simulink model "SimpleCalc_SF_Topic3_Task1"  (R2019a)
settings: Solver=FixedStepDiscrete  StartTime=0.0  StopTime=10.0  RelTol=1e-3
settings Model: Creator=Raouf  LastModifiedBy=Raouf
settings OptimizationCC: DefaultParameterBehavior=Inlined  EnhancedBackFolding=on  PassReuseOutputArgsAs=Individual arguments  OptimizeBlockOrder=speed  DifferentSizesBufferReuse=on  OptimizationCustomize=off
settings DebuggingCC: ParameterTunabilityLossMsg=error
settings SFSimCC: MATLABDynamicMemAlloc=off
settings RTWCC: SystemTargetFile=ert.tlc  GenCodeOnly=on  TemplateMakefile=ert_default_tmf  GenerateReport=on  IncludeHyperlinkInReport=on  LaunchReport=on  GenerateTraceInfo=on  GenerateTraceReport=on  GenerateTraceReportSl=on  GenerateTraceReportSf=on  GenerateTraceReportEml=on
settings CodeAppCC: ForceParamTrailComments=on  IgnoreCustomStorageClasses=off  OperatorAnnotations=on  SimulinkDataObjDesc=on  SFDataObjDesc=on  InsertBlockDesc=on
settings ERTTargetCC: TargetLangStandard=C99 (ISO)  GenerateSampleERTMain=on  InlinedParameterPlacement=NonHierarchical  ERTCustomFileTemplate=example_file_process.tlc

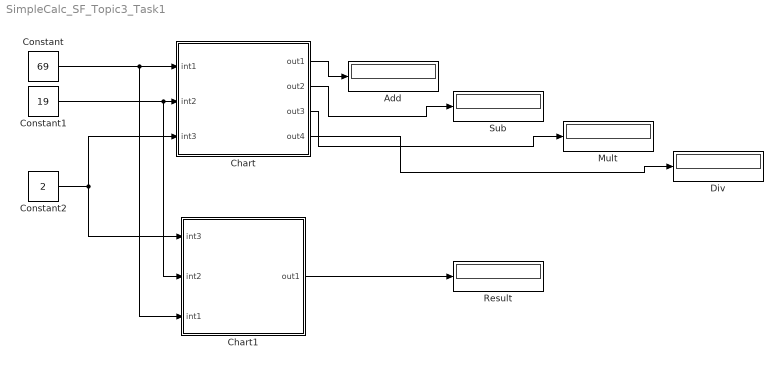
== system SimpleCalc_SF_Topic3_Task1 ==
  Add : Display
  Chart : Stateflow chart  TreatAsAtomicUnit=on
  Chart1 : Stateflow chart  BlockKeywords=__PRM__SERIALIZED__DATA__:Stateflow Chart,Stateflow Diagram  TreatAsAtomicUnit=on
  Constant : Constant  Value=69  OutDataTypeStr=int32
  Constant1 : Constant  Value=19  OutDataTypeStr=int32
  Constant2 : Constant  Value=2  OutDataTypeStr=int32
  Div : Display
  Mult : Display
  Result : Display
  Sub : Display
  wires:
  Chart/1(out1) -> Add/1
  Chart/2(out2) -> Sub/1
  Chart/3(out3) -> Mult/1
  Chart/4(out4) -> Div/1
  Constant/1 -> Chart/1(int1), Chart1/3(int1)
  Constant1/1 -> Chart1/2(int2), Chart/2(int2)
  Constant2/1 -> Chart/3(int3), Chart1/1(int3)
  Chart1/1(out1) -> Result/1

== stateflow chart SimpleCalc_SF_Topic3_Task1/Chart1 ==
  note: Do not put any code along
      | the transitions that run
      | down the right side!
  (default) -> (junction 27) : % calculator
  (junction 27) -> (junction 28) [order 1] : [int3 == 1]
  (junction 27) -> (junction 31) [order 2]
  (junction 28) -> (junction 29) : {out1 = int1 + int2;}
  (junction 29) -> (junction 30)
  (junction 30) -> (junction 34)
  (junction 31) -> (junction 32) [order 1] : [int3 == 2]
  (junction 31) -> (junction 35) [order 2]
  (junction 32) -> (junction 33) : {out1 = int1 - int2;}
  (junction 33) -> (junction 34)
  (junction 34) -> (junction 38)
  (junction 35) -> (junction 36) [order 1] : [int3 == 3]
  (junction 35) -> (junction 39) [order 2]
  (junction 36) -> (junction 37) : {out1 = int1 * int2;}
  (junction 37) -> (junction 38)
  (junction 38) -> (junction 42)
  (junction 39) -> (junction 40) [order 1] : [int3 == 4]
  (junction 39) -> (junction 43) [order 2] : {%Do Nothing
      | ;}
  (junction 40) -> (junction 41) : {out1 = int1 / int2;}
  (junction 41) -> (junction 42)
  (junction 42) -> (junction 44)
  (junction 44) -> (junction 43)
  (junction 43) -> (junction 45)
  data: out1 output int32; int3 input int32; int2 input int32; int1 input int32

== stateflow chart SimpleCalc_SF_Topic3_Task1/Chart ==
  state Sub
    out2 = int1 - int2;
  state Add
    out1 = int1 + int2;
  state Mult
    out3 = int1*int2;
  state SimpleCalculator
    entry:
    int1;
    int2;
    int3;
  note: Add
  note: Sub
  state Div
    out4 = int1/int2;
  (junction 12) -> Sub [order 2] : [int3 == 2]
  (junction 12) -> Add [order 1] : [int3 == 1]
  (default) -> SimpleCalculator
  (junction 12) -> Mult [order 3] : [int3 == 3]
  SimpleCalculator -> (junction 12)
  (junction 12) -> Div [order 4] : [int3 == 4]
  data: int1 input int32; int2 input int32; int3 input int32; out1 output int32; out2 output int32; out3 output int32; out4 output int32
